simulink model "Basic_Signal"  (R2024b)
settings: Solver=VariableStepAuto  StartTime=0.0  StopTime=10.0  RelTol=1e-3
libraries: simulink x2
settings Model: Creator=abdal  LastModifiedBy=abdal

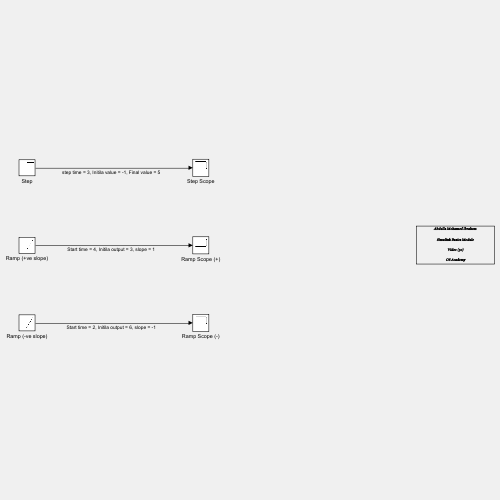
[thumbnail: Simulink's stored preview of the top-level diagram]
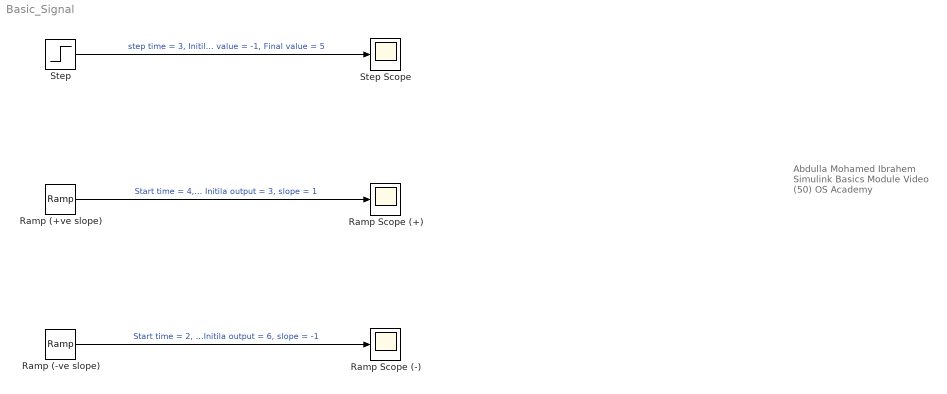
== system Basic_Signal ==
  note: Abdulla Mohamed Ibrahem
      | Simulink Basics Module
      | Video (50)
      | OS Academy
  Ramp (+ve slope) : simulink/Sources/Ramp  slope=1  start=4  InitialOutput=3
  Ramp (-ve slope) : simulink/Sources/Ramp  slope=-1  start=2  InitialOutput=6
  Ramp Scope (+) : Scope
  Ramp Scope (-) : Scope
  Step : Step  Time=3  Before=-1  After=5  SampleTime=0
  Step Scope : Scope
  wires:
  Step/1 -> Step Scope/1  "step time = 3, Initila value = -1, Final value = 5"
  Ramp (+ve slope)/1 -> Ramp Scope (+)/1  "Start time = 4, Initila output = 3, slope = 1"
  Ramp (-ve slope)/1 -> Ramp Scope (-)/1  "Start time = 2, Initila output = 6, slope = -1"
